simulink model "primer46_a"  (Simulink 6.3)
settings: Solver=ode45  StartTime=0.0  StopTime=4  RelTol=1e-3
settings Model: LastModifiedBy=GSGeorgiev

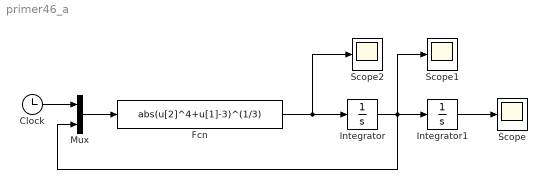
== system primer46_a ==
  Clock : Clock
      settings: Decimation=10
  Fcn : Fcn  Expr=abs(u[2]^4+u[1]-3)^(1/3)
  Integrator : Integrator  InitialCondition=-4
  Integrator1 : Integrator  InitialCondition=-5
  Mux : Mux  Inputs=2
  Scope : Scope
  Scope1 : Scope
  Scope2 : Scope
      settings: SaveName=ScopeData2
  wires:
  Clock/1 -> Mux/1
  Integrator/1 -> Integrator1/1, Scope1/1, Mux/2
  Fcn/1 -> Integrator/1, Scope2/1
  Mux/1 -> Fcn/1
  Integrator1/1 -> Scope/1
